simulink library "tqd"  (R2021b)
settings: Solver=VariableStepAuto  StartTime=0.0  StopTime=10.0  RelTol=1e-3
undefined symbols (not defined in the file): ATQD_AfterTqMinGain_X_Deg, ATQD_APSCreepBaseTqD_X_kph, ATQD_APSCreepBaseTqD_Y_Deg, ATQD_APSCreepBaseTqR_X_kph, ATQD_APSCreepBaseTqR_Y_Deg, ATQD_APSCreepIterm_X_kph, ATQD_APSCreepIterm_Y_kph, ATQD_APSCreepPterm_X_kph, ATQD_APSCreepPterm_Y_kph, ATQD_APSDecReq_X_kph, ATQD_APSDecReq_Y_mps2, ATQD_APSDecReqCMD_X_kph, ATQD_APSDecReqTs_X_pct, ATQD_APSDecTimeGain_X_Deg, ATQD_APSDecTimeGain_Y_s, ATQD_APSReqLowSpd_X_Deg, ATQD_AutoHoldReleaseBPS_X_Deg, ATQD_AWDLoadTrqnsGain_X_kg, ATQD_AWDLoadTrqnsGain_Y_pct, ATQD_BOSEnBPSPosn_X_kph, ATQD_BOSMap_X_rpm, ATQD_BOSMap_Y_pct, ATQD_CreepBaseTqD_X_kph, ATQD_CreepBaseTqD_Y_Deg, ATQD_CreepBaseTqR_X_kph, ATQD_CreepBaseTqR_Y_Deg, ATQD_CreepBPSDisPosn_X_Deg, ATQD_CreepBPSDisPosnR_X_Deg, ATQD_CreepBPSEnPosn_X_Deg, ATQD_CreepBPSEnPosnR_X_Deg, ATQD_CreepDeltaTq_X_kph, ATQD_CreepIterm_X_kph, ATQD_CreepIterm_Y_kph, ATQD_CreepItermMaxLimit_X_pct, ATQD_CreepPreloadTime_X_kph, ATQD_CreepPreloadTq_X_kph, ATQD_CreepPreloadTq_Y_s, ATQD_CreepProtTq_X_Deg, ATQD_CreepPterm_X_kph, ATQD_CreepPterm_Y_kph, ATQD_CreepRrTqSpRat_X_rpm, ATQD_CreepRrTqSpRat_Y_Nm, ATQD_CreepTargetSpdD_X_pct, ATQD_CreepTargetSpdR_X_pct, ATQD_ECOTqMapD_X_rpm, ATQD_ECOTqMapD_Y_pct, ATQD_EMTqMapD_X_rpm, ATQD_EMTqMapD_Y_pct, ATQD_EOPDTqMapDCon_X_rpm, ATQD_EOPDTqMapDCon_Y_Deg, ATQD_EscapeModePedTq_X_pct, ATQD_EscapeModePedTq_Y_rpm, ATQD_EscapeModePedTqFr_X_pct, ATQD_EscapeModePedTqFr_Y_rpm, ATQD_EstInitVehWeight_X_c, ATQD_FAfterTqCMDGain_X_rpm, ATQD_FAfterTqCMDGain_Y_pct, ATQD_FrLossMAPLowV_X_rpm, ATQD_FrLossMAPLowV_Y_Nm, ATQD_FrMotActReduce_X_rpm ... (+772)
libraries: simulink x211, hcu_lib x179, tqr x3
(part 6 of 28)

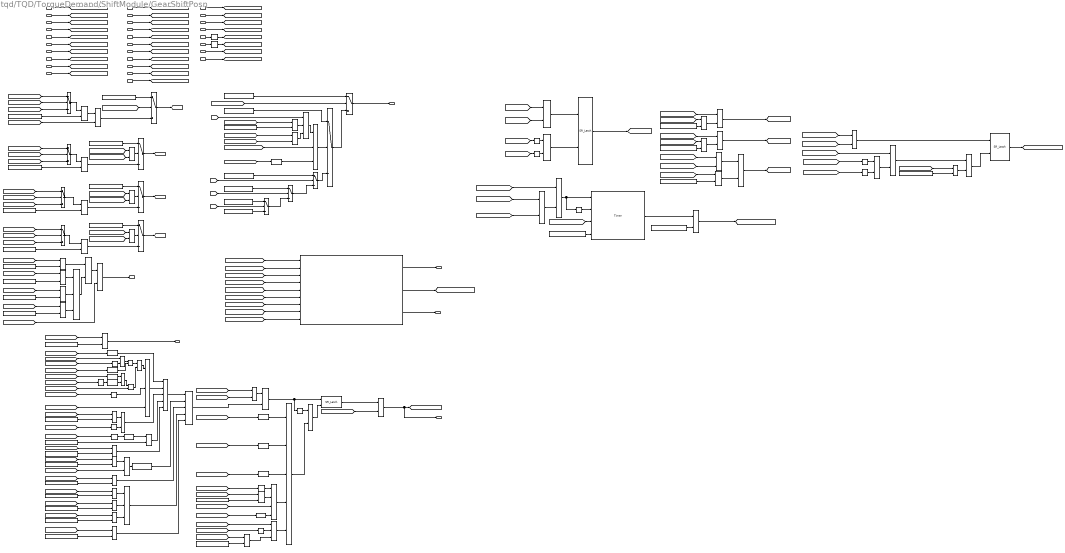
== system tqd/TQD/TorqueDemand/ShiftModule/GearShiftPosn ==
  note: Failsafe for Shifter PButton fail
  VTQD_ShifterHandleCmd_enum : Inport
  VPMM_PowerSta_enum : Inport  Port=2
  VINP_DrDoorSW_flg : Inport  Port=3
  VVMC_APSShiftPosnReq_enum : Inport  Port=4
  VVMC_APSActive_flg : Inport  Port=5
  VINP_DriverSeatBeltCmd_flg : Inport  Port=6
  VINP_SeatSW_flg : Inport  Port=7
  VTQD_EPBCarWashMode_flg : Inport  Port=8
  VTQD_VehActSpd_kph : Inport  Port=9
  VINP_ChrgPlugSta_enum : Inport  Port=10
  VTQD_GearActualPosn_enum : Inport  Port=11
  VTQD_AfterAvailableTqDemFr_Nm : Inport  Port=12
  VTQD_AfterAvailableTqDemRr_Nm : Inport  Port=13
  VTQR_NoABSFEDUWhlTqReq_Nm : Inport  Port=14
  VTQR_NoABSREDUWhlTqReq_Nm : Inport  Port=15
  task_time_s : Inport  Port=16
  VINP_DOASta_flg : Inport  Port=17
  VTQD_IVIPwrLock_flg : Inport  Port=18
  VTQD_BrkSwSta_flg : Inport  Port=19
  VTQD_OPDHoldAllowPark_flg : Inport  Port=20
  VINP_CAASSta_enum : Inport  Port=21
  VDDM_VCURAPSErrLv2_flg : Inport  Port=22
  VDDM_VCURAPSErrLv3_flg : Inport  Port=23
  VINP_APSStaSystem_enum : Inport  Port=24
  VDDM_Shifter1Err_flg : Inport  Port=25
  SWC_RegenUp : Inport  Port=26
  SWC_RegenDown : Inport  Port=27
  VDDM_ShifterSigErrCFS_flg : Inport  Port=28
  VTQD_ShifterFailsta_enum : Inport  Port=29
  AND{,1,6..9} (6 alike) : Logic  AllPortsSameDT=off  OutDataTypeStr=boolean
  AND2 : Logic  Inputs=4  AllPortsSameDT=off  OutDataTypeStr=boolean
  AND3 : Logic  Operator=OR  AllPortsSameDT=off  OutDataTypeStr=boolean
  AND4 : Logic  Inputs=3  AllPortsSameDT=off  OutDataTypeStr=boolean
  AND5 : Logic  Inputs=5  AllPortsSameDT=off  OutDataTypeStr=boolean
  Constant : Constant  Value=ENUM_GEARSHIFTCMD_R
  Constant1 : Constant  Value=ENUM_POWERSTA_READY
  Constant10 : Constant  Value=KTQD_OPDHoldAllowGearPSW_flg
  Constant11 : Constant  Value=ENUM_CAASSTA_SHIFTGEARTOP
  Constant12 : Constant  Value=ENUM_SHIFTCOMMAND_D
  Constant13 : Constant  Value=ENUM_SHIFTCOMMAND_N
  Constant14 : Constant  Value=ENUM_PWRSTASW_READY
  Constant15 : Constant  Value=ENUM_SHIFTCOMMAND_P
  Constant16 : Constant  Value=ENUM_CHRGPLUGSTA_NONE
  Constant17 : Constant  Value=ENUM_POWERSTA_STANDBY
  Constant18 : Constant  Value=ENUM_POWERSTA_ON
  Constant19 : Constant  Value=ENUM_POWERSTA_READY
  Constant2 : Constant  Value=ENUM_GEARSHIFTCMD_N
  Constant20 : Constant  Value=ENUM_APSSYSTEMSTA_REMOTEACTIVE
  Constant21 : Constant  Value=ENUM_APSSYSTEMSTA_REMOTEACTIVE
  Constant22 : Constant  Value=ENUM_CHRGPLUGSTA_NONE
  Constant23 : Constant  Value=ENUM_PWRSTASW_STANDBY
  Constant24 : Constant  Value=ENUM_PWRSTASW_ON
  Constant25 : Constant  Value=ENUM_PWRSTASW_READY
  Constant26 : Constant  Value=KTQD_ForcePLimitSpd_kph
  Constant27 : Constant  Value=KTQD_ShifterFail2P_s
  Constant28 : Constant  Value=KTQD_ShifterFail2P_s
  Constant29 : Constant  Value=KTQD_ForcePLimitSpd_kph
  Constant3 : Constant  Value=ENUM_GEARSHIFTCMD_P
  Constant30 : Constant  Value=ENUM_SHIFTERERRSTA_PBUTTONFAILURE
  Constant31 : Constant  Value=ENUM_SHIFTERERRSTA_HALLFAILURE
  Constant{5,32..34} (4 alike) : Constant  Value=FALSE
  Constant35 : Constant  Value=ENUM_SHIFTERERRSTA_SHIFTERFAILURE
  Constant36 : Constant  Value=ENUM_SHIFTCOMMAND_R
  Constant4 : Constant  Value=ENUM_GEARSHIFTCMD_D
  Constant6 : Constant  Value=ENUM_GEARSHIFTCMD_NONE
  Constant7 : Constant  Value=ENUM_GEARSHIFTCMD_P
  Constant8 : Constant  Value=ENUM_SHIFTCOMMAND_P
  Constant9 : Constant  Value=KTQD_DriveProtVehSpdGain_kph
  Delay{,1..3} (4 alike) : Delay  DelayLength=1
  Detect Change : simulink/Logic and Bit Operations/Detect Change  vinit=0  OutDataTypeStr=boolean
  Detect Change1 : simulink/Logic and Bit Operations/Detect Change  vinit=0  OutDataTypeStr=boolean
  Detect Decrease1 : simulink/Logic and Bit Operations/Detect Decrease  vinit=0.0  OutDataTypeStr=boolean
  Detect Increase{,1..6} (7 alike) : simulink/Logic and Bit Operations/Detect Increase  vinit=0.0  OutDataTypeStr=boolean
  Drive Protection : Subsystem
  Equal{,1..7,9..10,12..13,15..16,18..20} (17 alike) : RelationalOperator  Operator===  OutDataTypeStr=boolean  RndMeth=Simplest
  Equal11 : RelationalOperator  Operator=~=  OutDataTypeStr=boolean  RndMeth=Simplest
  Equal14 : RelationalOperator  Operator=~=  OutDataTypeStr=boolean  RndMeth=Simplest
  Equal8 : RelationalOperator  Operator=<=  OutDataTypeStr=boolean  RndMeth=Simplest
  Latch : hcu_lib/Basic_Blocks/Latch
  Logical Operator{,1,7,10..12,14,20,23} (9 alike) : Logic  AllPortsSameDT=off  OutDataTypeStr=boolean
      Logical Operator20 settings: AttributesFormatString=%<Operator>
  Logical Operator{8..9,13,16..19,24} (8 alike) : Logic  Operator=OR  AllPortsSameDT=off  OutDataTypeStr=boolean
      Logical Operator24 settings: AttributesFormatString=%<Operator>
  Logical Operator{4,15,21..22} (4 alike) : Logic  Operator=NOT  AllPortsSameDT=off  OutDataTypeStr=boolean
  Logical Operator2 : Logic  Inputs=3  AllPortsSameDT=off  OutDataTypeStr=boolean
  Logical Operator3 : Logic  Operator=OR  Inputs=3  AllPortsSameDT=off  OutDataTypeStr=boolean
  Logical Operator6 : Logic  Inputs=3  AllPortsSameDT=off  OutDataTypeStr=boolean
  NOT{,2..7} (7 alike) : Logic  Operator=NOT  AllPortsSameDT=off  OutDataTypeStr=boolean
  OR : Logic  Operator=OR  Inputs=3  AllPortsSameDT=off  OutDataTypeStr=boolean
  OR1 : Logic  Operator=OR  Inputs=5  AllPortsSameDT=off  OutDataTypeStr=boolean
  OR{2..6,9..10} (7 alike) : Logic  Operator=OR  AllPortsSameDT=off  OutDataTypeStr=boolean
  OR7 : Logic  Operator=OR  Inputs=5  AllPortsSameDT=off  OutDataTypeStr=boolean
  OR8 : Logic  Operator=OR  Inputs=3  AllPortsSameDT=off  OutDataTypeStr=boolean
  Relational Operator1 : RelationalOperator  Operator===  OutDataTypeStr=boolean  RndMeth=Simplest
  Relational Operator2 : RelationalOperator  Operator=<=  OutDataTypeStr=boolean  RndMeth=Simplest
  Relational Operator3 : RelationalOperator  OutDataTypeStr=boolean  RndMeth=Simplest
  Relational Operator4 : RelationalOperator  Operator=<=  OutDataTypeStr=boolean  RndMeth=Simplest
  Relational Operator5 : RelationalOperator  Operator=~=  OutDataTypeStr=boolean  RndMeth=Simplest
  SR_Latch : hcu_lib/Basic_Blocks/SR_Latch
  SR_Latch1 : hcu_lib/Basic_Blocks/SR_Latch
  SR_Latch3 : hcu_lib/Basic_Blocks/SR_Latch
  Switch{,1..4,7} (6 alike) : Switch  Criteria=u2 ~= 0
      Switch1 settings: AttributesFormatString=%<Criteria>
      Switch2 settings: AttributesFormatString=%<Criteria>
      Switch3 settings: AttributesFormatString=%<Criteria>
      Switch4 settings: AttributesFormatString=%<Criteria>
  Switch{5..6,8,10..13} (7 alike) : Switch  Criteria=u2 > Threshold
  Timer : hcu_lib/Basic_Blocks/Timer
  VTQD_GearShiftCMD_enum : Outport
  VTQD_PwrStaAllowPN_flg : Outport  Port=2
  VTQD_PwrStaAllowDR_flg : Outport  Port=3
  VTQD_DriveProtRemove_flg : Outport  Port=4
  VTQD_DriveProtEn_flg : Outport  Port=5
  VTQD_ForceP_flg : Outport  Port=6
  wires:
  Switch2/1 -> Switch4/3
  Constant2/1 -> Switch4/1
  Switch1/1 -> Switch2/3
  [P] -> Switch2/2
  Constant3/1 -> Switch2/1
  Switch3/1 -> Switch1/3
  Constant/1 -> Switch3/1
  Constant4/1 -> Switch1/1
  [R] -> Switch3/2
  [D] -> Switch1/2
  VTQD_ShifterHandleCmd_enum/1 -> [VTQD_ShifterHandleCmd_enum]
  Constant19/1 -> Equal6/2
  [VPMM_PowerSta_enum] -> Equal6/1
  [VPMM_PowerSta_enum] -> Equal5/1
  [VPMM_PowerSta_enum] -> Equal4/1
  Constant17/1 -> Equal4/2
  Constant18/1 -> Equal5/2
  VPMM_PowerSta_enum/1 -> [VPMM_PowerSta_enum]
  Equal5/1 -> OR/2
  Equal4/1 -> OR/1
  Equal6/1 -> OR/3
  [VPMM_PowerSta_enum] -> Equal7/1
  Constant1/1 -> Equal7/2
  Equal7/1 -> VTQD_PwrStaAllowDR_flg/1  "VTQD_PwrStaAllowDR_flg"
  Constant6/1 -> Switch3/3
  Switch/1 -> VTQD_GearShiftCMD_enum/1  "VTQD_GearShiftCMD_enum"
  Switch4/1 -> Switch/3
  VINP_DrDoorSW_flg/1 -> [VINP_DrDoorSW_flg]
  [VTQD_ForceP_flg] -> Switch/2
  Constant7/1 -> Switch/1
  VVMC_APSShiftPosnReq_enum/1 -> [VVMC_APSShiftPosnReq_enum]
  VVMC_APSActive_flg/1 -> [VVMC_APSActive_flg]
  VINP_SeatSW_flg/1 -> [VINP_SeatSW_flg]
  VINP_DriverSeatBeltCmd_flg/1 -> [VINP_DriverSeatBeltCmd_flg]
  VTQD_EPBCarWashMode_flg/1 -> [VTQD_EPBCarWashMode_flg]
  VTQD_VehActSpd_kph/1 -> [VTQD_VehActSpd_kph]
  VINP_ChrgPlugSta_enum/1 -> [VINP_ChrgPlugSta_enum]
  VTQR_NoABSREDUWhlTqReq_Nm/1 -> [VTQR_NoABSREDUWhlTqReq_Nm]
  VTQD_AfterAvailableTqDemFr_Nm/1 -> [VTQD_AfterAvailableTqDemFr_Nm]
  VTQD_GearActualPosn_enum/1 -> [VTQD_GearActualPosn_enum]
  VTQR_NoABSFEDUWhlTqReq_Nm/1 -> [VTQR_NoABSFEDUWhlTqReq_Nm]
  VTQD_AfterAvailableTqDemRr_Nm/1 -> [VTQD_AfterAvailableTqDemRr_Nm]
  task_time_s/1 -> [task_time_s]
  OR6/1 -> Logical Operator/1
  Logical Operator1/1 -> OR10/2
  [VTQD_EPBCarWashMode_flg] -> NOT4/1
  [VPMM_PowerSta_enum] -> Equal15/1
  [VTQD_VehActSpd_kph] -> Relational Operator2/1
  Logical Operator/1 -> OR10/1
  Detect Increase3/1 -> OR9/2
  [VINP_DrDoorSW_flg] -> Logical Operator1/2
  [VINP_SeatSW_flg] -> NOT5/1
  [VINP_DrDoorSW_flg] -> Detect Increase1/1
  OR9/1 -> Logical Operator1/1
  Detect Increase2/1 -> OR9/1
  Constant16/1 -> Equal14/2
  NOT5/1 -> Detect Increase3/1
  [VINP_DriverSeatBeltCmd_flg] -> Detect Increase2/1
  Equal12/1 -> OR8/2
  OR10/1 -> AND4/1
  AND4/1 -> OR7/2
  Equal15/1 -> OR8/1
  Constant23/1 -> Equal15/2
  Constant25/1 -> Equal13/2
  Detect Increase1/1 -> Logical Operator/2
  [VTQD_EPBCarWashMode_flg] -> Detect Decrease1/1
  Constant26/1 -> Relational Operator2/2
  [VPMM_PowerSta_enum] -> Equal13/1
  NOT4/1 -> AND4/2
  Constant24/1 -> Equal12/2
  Equal13/1 -> OR8/3
  [VINP_ChrgPlugSta_enum] -> Equal14/1
  OR7/1 -> AND5/1
  NOT3/1 -> OR6/2
  Detect Decrease1/1 -> OR7/1
  [VINP_DriverSeatBeltCmd_flg] -> OR6/1
  [VINP_SeatSW_flg] -> NOT3/1
  [VPMM_PowerSta_enum] -> Equal12/1
  VINP_DOASta_flg/1 -> [VINP_DOASta_flg]
  [VINP_DOASta_flg] -> AND4/3
  Constant9/1 -> Equal8/2
  [VTQD_VehActSpd_kph] -> Equal8/1
  [VTQD_EPBCarWashMode_flg] -> Detect Increase/1
  Detect Increase/1 -> Logical Operator3/3
  [N] -> Logical Operator2/1
  Logical Operator2/1 -> Logical Operator3/1
  Logical Operator3/1 -> Switch4/2
  [task_time_s] -> Drive Protection/8(task_time_s)  "task_time_s"
  [VTQD_VehActSpd_kph] -> Drive Protection/3(VTQD_VehActSpd_kph)
  [VTQD_AfterAvailableTqDemRr_Nm] -> Drive Protection/7(VTQD_AfterAvailableTqDemRr_Nm)
  Drive Protection/1(VTQD_DriveProtRemove_flg) -> VTQD_DriveProtRemove_flg/1
  [VTQD_AfterAvailableTqDemFr_Nm] -> Drive Protection/4(VTQD_AfterAvailableTqDemFr_Nm)
  [VTQR_NoABSREDUWhlTqReq_Nm] -> Drive Protection/5(VTQR_NoABSREDUWhlTqReq_Nm)
  [VTQR_NoABSFEDUWhlTqReq_Nm] -> Drive Protection/6(VTQR_NoABSFEDUWhlTqReq_Nm)
  [VTQD_ShifterHandleCmd_enum] -> Drive Protection/1(VTQD_ShifterHandleCmd_enum)
  Drive Protection/2(VTQD_DriveProtToPsnN_flg) -> [VTQD_DriveProtToPsnN_flg]
  [VTQD_GearActualPosn_enum] -> Drive Protection/2(VTQD_GearActualPosn_enum)
  VTQD_IVIPwrLock_flg/1 -> [VTQD_IVIPwrLock_flg]
  [VTQD_DriveProtToPsnN_flg] -> Logical Operator3/2
  Drive Protection/3(VTQD_DriveProtEn_flg) -> VTQD_DriveProtEn_flg/1
  [VTQD_IVIPwrLock_flg] -> OR2/2
  SR_Latch1/1 -> OR2/1
  OR2/1 -> VTQD_ForceP_flg/1, [VTQD_ForceP_flg]  "VTQD_ForceP_flg"
  [VPMM_PowerSta_enum] -> Equal3/1
  Latch/1 -> AND5/2
  Constant14/1 -> Equal3/2
  Relational Operator2/1 -> AND5/3
  OR8/1 -> AND5/4
  Equal8/1 -> Logical Operator2/2
  VTQD_BrkSwSta_flg/1 -> [VTQD_BrkSwSta_flg]
  [VTQD_BrkSwSta_flg] -> Drive Protection/9(VTQD_BrkSwSta_flg)
  OR3/1 -> Logical Operator2/3
  [VTQD_BrkSwSta_flg] -> OR3/1
  [VVMC_APSActive_flg] -> OR3/2
  VTQD_OPDHoldAllowPark_flg/1 -> [VTQD_OPDHoldAllowPark_flg]
  AND/1 -> OR7/4
  Detect Increase6/1 -> AND/1
  Constant10/1 -> AND/2
  [VTQD_OPDHoldAllowPark_flg] -> Delay/1
  Delay/1 -> Detect Increase6/1
  VINP_CAASSta_enum/1 -> [VINP_CAASSta_enum]
  [VINP_CAASSta_enum] -> Equal10/1
  Equal10/1 -> OR7/5
  Constant11/1 -> Equal10/2
  VDDM_VCURAPSErrLv3_flg/1 -> [VDDM_VCURAPSErrLv3_flg]
  VINP_APSStaSystem_enum/1 -> [VINP_APSStaSystem_enum]
  VDDM_VCURAPSErrLv2_flg/1 -> [VDDM_VCURAPSErrLv2_flg]
  [VVMC_APSActive_flg] -> Logical Operator7/1
  [VDDM_VCURAPSErrLv3_flg] -> Logical Operator7/2
  Logical Operator7/1 -> AND3/1
  AND5/1 -> AND3/2
  [VDDM_VCURAPSErrLv3_flg] -> Logical Operator4/1
  [VVMC_APSActive_flg] -> Detect Increase5/1
  [VINP_APSStaSystem_enum] -> Relational Operator1/1
  Logical Operator6/1 -> OR1/5
  Delay1/1 -> AND2/1
  Constant21/1 -> Relational Operator1/2
  [VTQD_ShifterHandleCmd_enum] -> Detect Change/1
  AND2/1 -> OR1/4
  Detect Increase5/1 -> OR1/3
  Equal11/1 -> AND2/2
  Detect Change1/1 -> AND2/4
  Relational Operator1/1 -> Logical Operator6/3
  [VVMC_APSShiftPosnReq_enum] -> Equal11/1
  [VTQD_EPBCarWashMode_flg] -> Detect Increase4/1
  [VDDM_VCURAPSErrLv2_flg] -> Logical Operator6/1
  OR1/1 -> AND1/2
  [VTQD_ForceP_flg] -> Delay1/1
  AND1/1 -> SR_Latch1/2
  Detect Increase4/1 -> OR1/2
  Detect Change/1 -> OR1/1
  [VVMC_APSShiftPosnReq_enum] -> Detect Change1/1
  Constant15/1 -> Equal11/2
  Logical Operator4/1 -> Logical Operator6/2
  [VVMC_APSActive_flg] -> AND2/3
  AND3/1 -> SR_Latch1/1, NOT/1
  NOT/1 -> AND1/1
  OR/1 -> AND6/2
  [VINP_ChrgPlugSta_enum] -> Equal16/1
  Constant22/1 -> Equal16/2
  Equal16/1 -> AND6/1
  AND6/1 -> OR4/1
  [VTQD_EPBCarWashMode_flg] -> OR4/2
  OR4/1 -> VTQD_PwrStaAllowPN_flg/1  "VTQD_PwrStaAllowPN_flg"
  Equal14/1 -> AND7/1
  [VTQD_EPBCarWashMode_flg] -> NOT2/1
  NOT2/1 -> AND7/2
  AND7/1 -> OR7/3
  Constant8/1 -> Equal/2
  Equal1/1 -> Switch11/3
  Switch8/1 -> Equal2/1
  Switch10/1 -> [P]
  [ShifterHall_Fail] -> Logical Operator17/1
  Constant33/1 -> Switch12/1
  [VVMC_APSShiftPosnReq_enum] -> Switch6/1
  [VVMC_APSActive_flg] -> Switch7/2
  [Shifter_Fail] -> Logical Operator18/2
  Switch13/1 -> [N]
  Constant13/1 -> Equal9/2
  [VVMC_APSActive_flg] -> Switch8/2
  [VVMC_APSShiftPosnReq_enum] -> Switch8/1
  [VVMC_APSActive_flg] -> Switch6/2
  Equal9/1 -> Switch13/3
  Logical Operator8/1 -> Switch11/2
  [Shifter_Fail] -> Logical Operator17/2
  Switch7/1 -> Equal9/1
  [VTQD_ShifterHandleCmd_enum] -> Switch5/3
  Constant5/1 -> Switch10/1
  Switch12/1 -> [D]
  [VVMC_APSShiftPosnReq_enum] -> Switch5/1
  Equal2/1 -> Switch12/3
  [VTQD_ShifterHandleCmd_enum] -> Switch6/3
  [VVMC_APSShiftPosnReq_enum] -> Switch7/1
  Constant12/1 -> Equal2/2
  Switch5/1 -> Equal/1
  Constant32/1 -> Switch11/1
  [ShifterHall_Fail] -> Logical Operator8/1
  Switch11/1 -> [R]
  Constant36/1 -> Equal1/2
  [VTQD_ShifterFail2P_flg] -> Logical Operator19/2
  [VTQD_ShifterHandleCmd_enum] -> Switch8/3
  [ShifterHall_Fail] -> Logical Operator18/1
  [VTQD_ShifterHandleCmd_enum] -> Switch7/3
  Equal/1 -> Logical Operator19/1
  Logical Operator19/1 -> Switch10/3
  Constant34/1 -> Switch13/1
  Logical Operator18/1 -> Switch13/2
  [VTQD_ShifterPBackUpCmd_flg] -> Switch10/2
  Switch6/1 -> Equal1/1
  [Shifter_Fail] -> Logical Operator8/2
  Logical Operator17/1 -> Switch12/2
  [VVMC_APSActive_flg] -> Switch5/2
  Logical Operator15/1 -> Timer/2
  [Shifter_Fail] -> Logical Operator16/2
  SR_Latch/1 -> [PRESS_BOTH]
  Constant29/1 -> Relational Operator4/2
  Logical Operator22/1 -> Logical Operator20/2
  AND9/1 -> SR_Latch/2
  Logical Operator13/1 -> Logical Operator14/1
  [VDDM_ShifterSigErrCFS_flg] -> Logical Operator12/1
  [VDDM_Shifter1Err_flg] -> Logical Operator13/2
  [SWC_RegenDown] -> NOT7/1
  Logical Operator21/1 -> Logical Operator20/1
  Logical Operator14/1 -> [Shifter_Fail]
  NOT7/1 -> AND9/2
  [task_time_s] -> Timer/3
  Relational Operator3/1 -> [VTQD_ShifterFail2P_flg]  "VTQD_ShifterFail2P_flg"
  [PRESS_BOTH] -> Logical Operator10/1
  Constant31/1 -> Equal19/2
  Logical Operator20/1 -> Logical Operator24/2
  [PRESS_BOTH] -> Logical Operator24/1
  Logical Operator12/1 -> [ShifterHall_Fail]
  [SWC_RegenUp] -> NOT6/1
  [Shifter_Fail] -> Logical Operator9/1
  [VTQD_ShifterFailsta_enum] -> Equal18/1
  Logical Operator16/1 -> SR_Latch3/1
  Logical Operator23/1 -> SR_Latch3/2
  Logical Operator24/1 -> Logical Operator23/1
  Relational Operator4/1 -> Logical Operator23/2
  [SWC_RegenDown] -> AND8/2
  [ShifterPButton_Fail] -> Logical Operator9/2
  Constant27/1 -> Timer/4
  Equal18/1 -> Logical Operator11/2
  Equal19/1 -> Logical Operator12/2
  [VDDM_ShifterSigErrCFS_flg] -> Logical Operator13/1
  [VDDM_ShifterSigErrCFS_flg] -> Logical Operator11/1
  AND8/1 -> SR_Latch/1
  Constant28/1 -> Relational Operator3/2
  Constant30/1 -> Equal18/2
  Timer/1 -> Relational Operator3/1
  Equal20/1 -> Logical Operator14/2
  Logical Operator9/1 -> Logical Operator10/2
  SR_Latch3/1 -> [VTQD_ShifterPBackUpCmd_flg]
  [ShifterPButton_Fail] -> Logical Operator16/1
  Logical Operator11/1 -> [ShifterPButton_Fail]
  [SWC_RegenUp] -> AND8/1
  [VTQD_ShifterFailsta_enum] -> Equal19/1
  Constant35/1 -> Equal20/2
  [VTQD_VehActSpd_kph] -> Relational Operator4/1
  NOT6/1 -> AND9/1
  [VTQD_ShifterFailsta_enum] -> Equal20/1
  Logical Operator10/1 -> Logical Operator15/1, Timer/1
  [VDDM_Shifter1Err_flg] -> Logical Operator22/1
  [VDDM_ShifterSigErrCFS_flg] -> Logical Operator21/1
  Constant20/1 -> Relational Operator5/2
  [VINP_APSStaSystem_enum] -> Relational Operator5/1
  Relational Operator5/1 -> AND5/5
  VDDM_ShifterSigErrCFS_flg/1 -> [VDDM_ShifterSigErrCFS_flg]
  Delay2/1 -> [SWC_RegenUp]
  SWC_RegenUp/1 -> Delay2/1
  Delay3/1 -> [SWC_RegenDown]
  SWC_RegenDown/1 -> Delay3/1
  VDDM_Shifter1Err_flg/1 -> [VDDM_Shifter1Err_flg]
  VTQD_ShifterFailsta_enum/1 -> [VTQD_ShifterFailsta_enum]
  [VINP_DOASta_flg] -> OR5/2
  Equal3/1 -> OR5/1
  OR5/1 -> Latch/1

== system tqd/TQD/TorqueDemand/ShiftModule/P_Button_State_Judge ==
  VTQD_ShifterHandleCmd_enum : Inport
  VVMC_APSActive_flg : Inport  Port=2
  VVMC_APSShiftPosnReq_enum : Inport  Port=3
  VTQD_ParkRequest_flg : Inport  Port=4
  VINP_EPBSta_enum : Inport  Port=5
  AND : Logic  AllPortsSameDT=off  OutDataTypeStr=boolean
  AND1 : Logic  Operator=OR  AllPortsSameDT=off  OutDataTypeStr=boolean
  Constant1 : Constant  Value=ENUM_PBUTTON_RELEASED
  Constant10 : Constant  Value=ENUM_EPBSTA_APPLIED
  Constant12 : Constant  Value=ENUM_SHIFTCOMMAND_D
  Constant15 : Constant  Value=ENUM_SHIFTCOMMAND_N
  Constant2 : Constant  Value=ENUM_PBUTTON_PRESSED
  Constant3 : Constant  Value=ENUM_PBUTTON_INVALID
  Constant4 : Constant  Value=ENUM_SHIFTCOMMAND_NONE
  Constant5 : Constant  Value=ENUM_SHIFTCOMMAND_P
  Constant6 : Constant  Value=ENUM_SHIFTCOMMAND_P
  Constant7 : Constant  Value=ENUM_PBUTTON_PRESSED
  Constant8 : Constant  Value=ENUM_SHIFTCOMMAND_R
  Constant9 : Constant  Value=ENUM_EPBSTA_APPLIED
  Detect Decrease : simulink/Logic and Bit Operations/Detect Decrease  vinit=boolean(0)  OutDataTypeStr=boolean
  Detect Decrease1 : simulink/Logic and Bit Operations/Detect Decrease  vinit=boolean(0)  OutDataTypeStr=boolean
  Detect Increase : simulink/Logic and Bit Operations/Detect Increase  vinit=boolean(0)  OutDataTypeStr=boolean
  Detect Increase1 : simulink/Logic and Bit Operations/Detect Increase  vinit=boolean(0)  OutDataTypeStr=boolean
  Equal{,1..7} (8 alike) : RelationalOperator  Operator===  OutDataTypeStr=boolean  RndMeth=Simplest
  Logical Operator : Logic  Operator=OR  Inputs=4  AllPortsSameDT=off  OutDataTypeStr=boolean
  NOT : Logic  Operator=NOT  AllPortsSameDT=off  OutDataTypeStr=boolean
  OR : Logic  Operator=OR  AllPortsSameDT=off  OutDataTypeStr=boolean
  OR1 : Logic  Operator=OR  Inputs=3  AllPortsSameDT=off  OutDataTypeStr=boolean
  SR_Latch : hcu_lib/Basic_Blocks/SR_Latch
  SR_Latch1 : hcu_lib/Basic_Blocks/SR_Latch
  Switch1 : Switch  Criteria=u2 ~= 0
      settings: AttributesFormatString=%<Criteria>
  Switch2 : Switch  Criteria=u2 ~= 0
      settings: AttributesFormatString=%<Criteria>
  Switch4 : Switch  Criteria=u2 ~= 0
      settings: AttributesFormatString=%<Criteria>
  VTQD_PButtonSta_enum : Outport
  wires:
  VTQD_ShifterHandleCmd_enum/1 -> [VTQD_ShifterHandleCmd_enum]
  Equal/1 -> [P]
  Constant12/1 -> Equal2/2
  [VTQD_ShifterHandleCmd_enum] -> Equal1/1
  Constant8/1 -> Equal1/2
  [VTQD_ShifterHandleCmd_enum] -> Equal/1
  Equal2/1 -> Logical Operator/3
  Constant15/1 -> Equal3/2
  Equal3/1 -> Logical Operator/2
  Equal1/1 -> Logical Operator/1
  Constant5/1 -> Equal/2
  [VTQD_ShifterHandleCmd_enum] -> Equal3/1
  [VTQD_ShifterHandleCmd_enum] -> Equal2/1
  Logical Operator/1 -> [RND]
  [RND] -> Switch4/2
  [P] -> Switch1/2
  Constant1/1 -> Switch4/1
  Switch1/1 -> Switch4/3
  Constant2/1 -> Switch1/1
  Constant3/1 -> Switch1/3
  [VTQD_ShifterHandleCmd_enum] -> Equal4/1
  Constant4/1 -> Equal4/2
  Equal4/1 -> Logical Operator/4
  Switch4/1 -> Switch2/3
  VVMC_APSActive_flg/1 -> [VVMC_APSActive_flg]
  VVMC_APSShiftPosnReq_enum/1 -> [VVMC_APSShiftPosnReq_enum]
  Switch2/1 -> VTQD_PButtonSta_enum/1  "VTQD_PButtonSta_enum"
  [VVMC_APSShiftPosnReq_enum] -> Equal5/1
  Constant6/1 -> Equal5/2
  [VVMC_APSActive_flg] -> AND/1
  Equal5/1 -> AND/2
  Constant7/1 -> Switch2/1
  VTQD_ParkRequest_flg/1 -> [VTQD_ParkRequest_flg]
  AND1/1 -> Switch2/2
  SR_Latch/1 -> AND1/1
  [VTQD_ParkRequest_flg] -> Detect Decrease/1, Detect Increase/1
  [VINP_EPBSta_enum] -> Equal6/1
  Detect Increase/1 -> SR_Latch/1
  Constant9/1 -> Equal6/2
  VINP_EPBSta_enum/1 -> [VINP_EPBSta_enum]
  OR/1 -> SR_Latch/2
  Equal6/1 -> OR/2
  Detect Decrease/1 -> OR/1
  AND/1 -> Detect Decrease1/1, Detect Increase1/1
  Detect Increase1/1 -> SR_Latch1/1
  [VINP_EPBSta_enum] -> Equal7/1
  Constant10/1 -> Equal7/2
  OR1/1 -> SR_Latch1/2
  SR_Latch1/1 -> AND1/2
  Equal7/1 -> OR1/3
  Detect Decrease1/1 -> OR1/1
  NOT/1 -> OR1/2
  [VVMC_APSActive_flg] -> NOT/1

== system tqd/TQD/TorqueDemand/ShiftModule/SR_Latch1 ==
  set : Inport
  reset : Inport  Port=2
  Logical Operator : Logic  AllPortsSameDT=off  OutDataTypeStr=boolean
  Logical Operator1 : Logic  Operator=NOT  AllPortsSameDT=off  OutDataTypeStr=boolean
  Switch1 : Switch  Criteria=u2 ~= 0  Threshold=0.5
      settings: AttributesFormatString=<Criteria=%<Criteria>>
  Switch2 : Switch  Criteria=u2 ~= 0  Threshold=0.5
      settings: AttributesFormatString=<Criteria=%<Criteria>>
  Unit Delay : UnitDelay  SampleTime=-1  HasFrameUpgradeWarning=on
  latched : Outport
  wires:
  Switch1/1 -> Unit Delay/1, latched/1
  set/1 -> Switch1/1, Logical Operator/1
  reset/1 -> Switch2/2, Logical Operator1/1
  Unit Delay/1 -> Switch2/3
  Switch2/1 -> Switch1/3
  Logical Operator/1 -> Switch1/2
  Logical Operator1/1 -> Logical Operator/2, Switch2/1

== system tqd/TQD/TorqueDemand/Signal_convert/AWDMCUReadyExt_flg ==
  VINP_FrMCUErr_enum : Inport
  VINP_RrMCUErr_enum : Inport  Port=2
  Action Port : ActionPort
  Constant : Constant  Value=ENUM_MCUWARN_LV0
  Constant1 : Constant  Value=ENUM_MCUWARN_NOERROR
  Constant2 : Constant  Value=ENUM_MCUWARN_LV0
  Constant3 : Constant  Value=ENUM_MCUWARN_NOERROR
  Equal{,1..3} (4 alike) : RelationalOperator  Operator===  OutDataTypeStr=boolean  RndMeth=Simplest
  Logical Operator : Logic  Operator=OR  AllPortsSameDT=off  OutDataTypeStr=boolean
  Logical Operator1 : Logic  Operator=OR  AllPortsSameDT=off  OutDataTypeStr=boolean
  Logical Operator2 : Logic  AllPortsSameDT=off  OutDataTypeStr=boolean
  VTQD_AWDMCUReadyExt_flg : Outport
  wires:
  Logical Operator2/1 -> VTQD_AWDMCUReadyExt_flg/1
  Equal1/1 -> Logical Operator/2
  Equal/1 -> Logical Operator/1
  Constant1/1 -> Equal1/2
  VINP_FrMCUErr_enum/1 -> Equal1/1, Equal/1
  Constant/1 -> Equal/2
  Equal3/1 -> Logical Operator1/2
  Equal2/1 -> Logical Operator1/1
  Constant3/1 -> Equal3/2
  VINP_RrMCUErr_enum/1 -> Equal3/1, Equal2/1
  Constant2/1 -> Equal2/2
  Logical Operator/1 -> Logical Operator2/1
  Logical Operator1/1 -> Logical Operator2/2

== system tqd/TQD/TorqueDemand/Signal_convert/FWDMCUReadyExt_flg ==
  VINP_FrMCUErr_enum : Inport
  Action Port : ActionPort
  Constant : Constant  Value=ENUM_MCUWARN_LV0
  Constant1 : Constant  Value=ENUM_MCUWARN_NOERROR
  Equal : RelationalOperator  Operator===  OutDataTypeStr=boolean  RndMeth=Simplest
  Equal1 : RelationalOperator  Operator===  OutDataTypeStr=boolean  RndMeth=Simplest
  Logical Operator : Logic  Operator=OR  AllPortsSameDT=off  OutDataTypeStr=boolean
  VTQD_FWDMCUReadyExt_flg : Outport
  wires:
  Logical Operator/1 -> VTQD_FWDMCUReadyExt_flg/1
  Equal/1 -> Logical Operator/1
  VINP_FrMCUErr_enum/1 -> Equal1/1, Equal/1
  Constant/1 -> Equal/2
  Constant1/1 -> Equal1/2
  Equal1/1 -> Logical Operator/2

== system tqd/TQD/TorqueDemand/Signal_convert/New Wheel Slide Rate ==
  VINP_LFRawWhlSpeed_kph : Inport
  VINP_LRRawWhlSpeed_kph : Inport  Port=2
  VINP_RFRawWhlSpeed_kph : Inport  Port=3
  VINP_RRRawWhlSpeed_kph : Inport  Port=4
  VINP_VehSpeed_kph : Inport  Port=5
  task_time_s : Inport  Port=6
  VTQR_NoABSFEDUWhlTqReq_Nm : Inport  Port=7
  VTQR_NoABSREDUWhlTqReq_Nm : Inport  Port=8
  Abs{,1..7} (8 alike) : Abs
  Add : Sum
  Add{1..4} (4 alike) : Sum  Inputs=+-
  Constant{1,4,6,9,11,15,18,135} (8 alike) : Constant  Value=eps
  Constant{5,10,14,128} (4 alike) : Constant  Value=KTQD_NewSlideRateTs_c
  Constant{2,7,12,16,19} (5 alike) : Constant  Value=ZERO_FLOAT
  Constant{3,8,13,17} (4 alike) : Constant  Value=ONE_PERCENT
  Data Type Conversion{,1..3} (4 alike) : DataTypeConversion  OutDataTypeStr=single
  Delay : Delay  DelayLength=1
  Delay1 : Delay  DelayLength=1
  Divide{,1..7} (8 alike) : Product  Inputs=*/
  FirstOrderFilter{,1..3} (4 alike) : hcu_lib/Basic_Blocks/FirstOrderFilter
  Max{,1..3} (4 alike) : MinMax  Function=max  Inputs=2
  Max4 : MinMax  Function=max  Inputs=4
  Max5 : MinMax  Inputs=4
  Min : MinMax  Inputs=5
  Relational Operator{,1..3} (4 alike) : RelationalOperator  Operator=<=  OutDataTypeStr=boolean  RndMeth=Simplest
  Relational Operator{4..7} (4 alike) : RelationalOperator  OutDataTypeStr=boolean  RndMeth=Simplest
  Relational Operator8 : RelationalOperator  Operator=>  OutDataTypeStr=boolean  RndMeth=Simplest
  Switch{,1..8} (9 alike) : Switch  Criteria=u2 > Threshold
  VTQD_MaxWhlSlideRate_pct : Outport
  VTQD_MinWhlSlideRate_pct : Outport  Port=2
  VTQD_LeftSlideRate_pct : Outport  Port=3
  VTQD_RightSlideRate_pct : Outport  Port=4
  VTQD_FrontSlideRate_pct : Outport  Port=5
  VTQD_RearSlideRate_pct : Outport  Port=6
  VTQD_LFSlideRate_pct : Outport  Port=7
  VTQD_LRSlideRate_pct : Outport  Port=8
  VTQD_RFSlideRate_pct : Outport  Port=9
  VTQD_RRSlideRate_pct : Outport  Port=10
  wires:
  [VTQD_RRSlideRate_pct] -> Max4/4
  Divide3/1 -> Switch1/3
  [task_time_s] -> FirstOrderFilter2/2
  [VTQD_FrontSlideRate_pct] -> VTQD_FrontSlideRate_pct/1
  FirstOrderFilter3/1 -> Divide6/1
  Switch4/1 -> [VTQD_LeftSlideRate_pct]  "VTQD_LeftSlideRate_pct"
  Add4/1 -> Divide7/1
  Switch5/1 -> [VTQD_RightSlideRate_pct]  "VTQD_RightSlideRate_pct"
  task_time_s/1 -> [task_time_s]
  [VTQD_LRSlideRate_pct] -> Abs6/1
  FirstOrderFilter1/1 -> Divide2/1
  Divide1/1 -> Switch/3
  Switch6/1 -> [VTQD_FrontSlideRate_pct]  "VTQD_FrontSlideRate_pct"
  Max4/1 -> [VTQD_MaxWhlSlideRate_pct]  "VTQD_MaxWhlSlideRate_pct"
  Constant17/1 -> Divide6/2
  Constant10/1 -> FirstOrderFilter2/3
  [VTQD_LFSlideRate_pct] -> Abs4/1
  Relational Operator4/1 -> Switch4/2
  Max/1 -> Divide1/2
  [VTQD_VehSpeed4Cal_kph] -> Relational Operator3/1
  [VTQD_LRSlideRate_pct] -> Max4/2
  FirstOrderFilter2/1 -> Divide4/1
  Constant13/1 -> Divide4/2
  Divide6/1 -> [VTQD_RRSlideRate_pct]  "VTQD_RRSlideRate_pct"
  Relational Operator6/1 -> Switch6/2
  [VTQD_LFSlideRate_pct] -> Abs/1
  Switch3/1 -> FirstOrderFilter3/1
  [VTQD_LeftSlideRate_pct] -> VTQD_LeftSlideRate_pct/1
  [VTQD_VehSpeed4Cal_kph] -> Max3/1
  [VTQD_RFSlideRate_pct] -> Max5/3
  [VTQD_VehSpeed4Cal_kph] -> Add4/2
  Relational Operator7/1 -> Switch7/2
  Abs5/1 -> Relational Operator6/2
  [task_time_s] -> FirstOrderFilter3/2
  [VINP_RFRawWhlSpeed_kph] -> Add3/1
  Constant14/1 -> FirstOrderFilter3/3
  [VTQD_RRSlideRate_pct] -> Switch7/3
  [task_time_s] -> FirstOrderFilter1/2
  Switch2/1 -> FirstOrderFilter2/1
  Abs6/1 -> Relational Operator7/1
  Constant16/1 -> Switch3/1
  [VTQD_RearSlideRate_pct] -> VTQD_RearSlideRate_pct/1
  Constant18/1 -> Relational Operator3/2
  Max3/1 -> Divide7/2
  Switch7/1 -> [VTQD_RearSlideRate_pct]  "VTQD_RearSlideRate_pct"
  Relational Operator3/1 -> Switch3/2
  [VTQD_LFSlideRate_pct] -> Switch6/1
  Abs/1 -> Relational Operator4/1
  [VTQD_VehSpeed4Cal_kph] -> Relational Operator2/1
  VINP_RFRawWhlSpeed_kph/1 -> [VINP_RFRawWhlSpeed_kph]
  Abs7/1 -> Relational Operator7/2
  Divide/1 -> [VTQD_LFSlideRate_pct]  "VTQD_LFSlideRate_pct"
  [VTQD_RRSlideRate_pct] -> Abs7/1
  Constant2/1 -> Switch/1
  Divide7/1 -> Switch3/3
  [VTQD_LRSlideRate_pct] -> Switch7/1
  Abs1/1 -> Relational Operator4/2
  Relational Operator2/1 -> Switch2/2
  [VTQD_RightSlideRate_pct] -> VTQD_RightSlideRate_pct/1
  [task_time_s] -> FirstOrderFilter/2
  Constant3/1 -> Divide/2
  [VTQD_RFSlideRate_pct] -> Switch6/3
  [VTQD_VehSpeed4Cal_kph] -> Add2/2
  Divide2/1 -> [VTQD_LRSlideRate_pct]  "VTQD_LRSlideRate_pct"
  [VINP_LFRawWhlSpeed_kph] -> Add2/1
  [VTQD_RFSlideRate_pct] -> Abs5/1
  Abs4/1 -> Relational Operator6/1
  VINP_RRRawWhlSpeed_kph/1 -> [VINP_RRRawWhlSpeed_kph]
  Constant9/1 -> Relational Operator2/2
  Constant12/1 -> Switch2/1
  Divide4/1 -> [VTQD_RFSlideRate_pct]  "VTQD_RFSlideRate_pct"
  [VTQD_LRSlideRate_pct] -> Switch4/3
  [VTQD_MinWhlSlideRate_pct] -> VTQD_MinWhlSlideRate_pct/1
  [VTQD_LRSlideRate_pct] -> Max5/2
  [VTQD_RRSlideRate_pct] -> Max5/4
  Max5/1 -> [VTQD_MinWhlSlideRate_pct]  "VTQD_MinWhlSlideRate_pct"
  Constant128/1 -> FirstOrderFilter/3
  [VTQD_LFSlideRate_pct] -> Max5/1
  Abs3/1 -> Relational Operator5/2
  [VTQD_VehSpeed4Cal_kph] -> Max/1
  [VINP_LRRawWhlSpeed_kph] -> Add1/1
  Relational Operator5/1 -> Switch5/2
  [VTQD_RRSlideRate_pct] -> Switch5/3
  [VTQD_RFSlideRate_pct] -> Switch5/1
  Abs2/1 -> Relational Operator5/1
  [VTQD_RRSlideRate_pct] -> Abs3/1
  [VTQD_RFSlideRate_pct] -> Abs2/1
  Constant8/1 -> Divide2/2
  Add2/1 -> Divide1/1
  Constant7/1 -> Switch1/1
  Relational Operator1/1 -> Switch1/2
  Max1/1 -> Divide3/2
  Constant5/1 -> FirstOrderFilter1/3
  Constant4/1 -> Relational Operator1/2
  Switch1/1 -> FirstOrderFilter1/1
  [VTQD_VehSpeed4Cal_kph] -> Relational Operator1/1
  [VTQD_VehSpeed4Cal_kph] -> Max1/1
  Add1/1 -> Divide3/1
  [VTQD_VehSpeed4Cal_kph] -> Add1/2
  VINP_LFRawWhlSpeed_kph/1 -> [VINP_LFRawWhlSpeed_kph]
  Relational Operator/1 -> Switch/2
  [VTQD_VehSpeed4Cal_kph] -> Relational Operator/1
  Constant1/1 -> Relational Operator/2
  [VTQD_LRSlideRate_pct] -> Abs1/1
  VINP_VehSpeed_kph/1 -> [VINP_VehSpeed_kph]
  VINP_LRRawWhlSpeed_kph/1 -> [VINP_LRRawWhlSpeed_kph]
  [VTQD_RFSlideRate_pct] -> Max4/3
  [VTQD_MaxWhlSlideRate_pct] -> VTQD_MaxWhlSlideRate_pct/1
  [VINP_RRRawWhlSpeed_kph] -> Add4/1
  FirstOrderFilter/1 -> Divide/1
  Switch/1 -> FirstOrderFilter/1
  [VTQD_LFSlideRate_pct] -> Switch4/1
  [VTQD_LFSlideRate_pct] -> Max4/1
  [VTQD_VehSpeed4Cal_kph] -> Add3/2
  [VTQD_VehSpeed4Cal_kph] -> Max2/1
  Add3/1 -> Divide5/1
  Max2/1 -> Divide5/2
  Divide5/1 -> Switch2/3
  Constant11/1 -> Data Type Conversion/1
  Data Type Conversion/1 -> Max2/2
  Data Type Conversion1/1 -> Max1/2
  Constant6/1 -> Data Type Conversion1/1
  Data Type Conversion2/1 -> Max/2
  Constant135/1 -> Data Type Conversion2/1
  Data Type Conversion3/1 -> Max3/2
  Constant15/1 -> Data Type Conversion3/1
  VTQR_NoABSFEDUWhlTqReq_Nm/1 -> [VTQR_NoABSFEDUWhlTqReq_Nm]
  VTQR_NoABSREDUWhlTqReq_Nm/1 -> [VTQR_NoABSREDUWhlTqReq_Nm]
  Add/1 -> Relational Operator8/1
  [VINP_VehSpeed_kph] -> Switch8/3
  Constant19/1 -> Relational Operator8/2
  Relational Operator8/1 -> Switch8/2
  Min/1 -> Switch8/1
  [VINP_LFRawWhlSpeed_kph] -> Min/1
  [VINP_LRRawWhlSpeed_kph] -> Min/2
  [VINP_RFRawWhlSpeed_kph] -> Min/3
  [VINP_RRRawWhlSpeed_kph] -> Min/4
  [VINP_VehSpeed_kph] -> Min/5
  [VTQR_NoABSFEDUWhlTqReq_Nm] -> Delay/1
  Delay/1 -> Add/1
  Delay1/1 -> Add/2
  [VTQR_NoABSREDUWhlTqReq_Nm] -> Delay1/1
  Switch8/1 -> [VTQD_VehSpeed4Cal_kph]  "VTQD_VehSpeed4Cal_kph"
  [VTQD_LRSlideRate_pct] -> VTQD_LRSlideRate_pct/1
  [VTQD_RRSlideRate_pct] -> VTQD_RRSlideRate_pct/1
  [VTQD_LFSlideRate_pct] -> VTQD_LFSlideRate_pct/1
  [VTQD_RFSlideRate_pct] -> VTQD_RFSlideRate_pct/1

== system tqd/TQD/TorqueDemand/Signal_convert/OUTPUT ONLY ON or READY ==
  note: INPUT Signals
  VPMM_PowerSta_enum : Inport
  VTQD_SWCRegenUpSta_flg : Inport  Port=2
  VTQD_SWCRegenDownSta_flg : Inport  Port=3
  VINP_ADASACCSta_enum : Inport  Port=4
  VVMC_CCCtrlSta_enum : Inport  Port=5
  VBCM_BrakeLamp_flg : Inport  Port=6
  VINP_VehSpeed_kph : Inport  Port=7
  AND : Logic  Inputs=6  AllPortsSameDT=off  OutDataTypeStr=boolean
  Constant1 : Constant  Value=ENUM_ADASACCSTA_ACTIVE
  Constant10 : Constant  Value=FALSE
  Constant11 : Constant  Value=KTQD_RegenButEnSpd_kph
  Constant3 : Constant  Value=ENUM_POWERSTA_ON
  Constant5 : Constant  Value=FALSE
  Constant6 : Constant  Value=ENUM_ADASACCSTA_OVERRIDE
  Constant7 : Constant  Value=ENUM_POWERSTA_READY
  Constant8 : Constant  Value=ENUM_ADASCCSTA_ACTIVE
  Constant9 : Constant  Value=ENUM_ADASCCSTA_OVRRIDE
  Equal2 : RelationalOperator  Operator===  OutDataTypeStr=boolean  RndMeth=Simplest
  Equal3 : RelationalOperator  Operator===  OutDataTypeStr=boolean  RndMeth=Simplest
  Equal{4..7} (4 alike) : RelationalOperator  Operator=~=  OutDataTypeStr=boolean  RndMeth=Simplest
  NOT : Logic  Operator=NOT  AllPortsSameDT=off  OutDataTypeStr=boolean
  OR1 : Logic  Operator=OR  AllPortsSameDT=off  OutDataTypeStr=boolean
  OR2 : Logic  Operator=OR  AllPortsSameDT=off  OutDataTypeStr=boolean
  Relational Operator : RelationalOperator  Operator=<=  OutDataTypeStr=boolean  RndMeth=Simplest
  Switch : Switch  Criteria=u2 ~= 0
  Switch1 : Switch  Criteria=u2 ~= 0
  SWC_RegenUp : Outport
  SWC_RegenDown : Outport  Port=2
  wires:
  Constant5/1 -> Switch/3
  Switch/1 -> SWC_RegenUp/1  "SWC_RegenUp"
  VTQD_SWCRegenUpSta_flg/1 -> Switch/1
  VTQD_SWCRegenDownSta_flg/1 -> Switch1/1
  Switch1/1 -> SWC_RegenDown/1  "SWC_RegenDown"
  Constant10/1 -> Switch1/3
  AND/1 -> Switch1/2, Switch/2
  VPMM_PowerSta_enum/1 -> [VPMM_PowerSta_enum]
  VINP_ADASACCSta_enum/1 -> [VINP_ADASACCSta_enum]
  VVMC_CCCtrlSta_enum/1 -> [VVMC_CCCtrlSta_enum]
  VBCM_BrakeLamp_flg/1 -> [VBCM_BrakeLamp_flg]
  VINP_VehSpeed_kph/1 -> [VINP_VehSpeed_kph]
  Relational Operator/1 -> OR2/2
  NOT/1 -> OR2/1
  OR2/1 -> AND/6
  Constant11/1 -> Relational Operator/2
  [VINP_VehSpeed_kph] -> Relational Operator/1
  Equal4/1 -> AND/2
  Equal5/1 -> AND/3
  Equal6/1 -> AND/4
  Equal7/1 -> AND/5
  OR1/1 -> AND/1
  Constant8/1 -> Equal6/2
  Constant9/1 -> Equal7/2
  [VBCM_BrakeLamp_flg] -> NOT/1
  [VVMC_CCCtrlSta_enum] -> Equal7/1
  [VVMC_CCCtrlSta_enum] -> Equal6/1
  [VINP_ADASACCSta_enum] -> Equal5/1
  Constant6/1 -> Equal5/2
  Constant1/1 -> Equal4/2
  [VINP_ADASACCSta_enum] -> Equal4/1
  Equal3/1 -> OR1/2
  [VPMM_PowerSta_enum] -> Equal2/1
  Constant7/1 -> Equal3/2
  Constant3/1 -> Equal2/2
  Equal2/1 -> OR1/1
  [VPMM_PowerSta_enum] -> Equal3/1

== system tqd/TQD/TorqueDemand/Signal_convert/RWDMCUReadyExt_flg ==
  VINP_RrMCUErr_enum : Inport
  Action Port : ActionPort
  Constant : Constant  Value=ENUM_MCUWARN_LV0
  Constant1 : Constant  Value=ENUM_MCUWARN_NOERROR
  Equal : RelationalOperator  Operator===  OutDataTypeStr=boolean  RndMeth=Simplest
  Equal1 : RelationalOperator  Operator===  OutDataTypeStr=boolean  RndMeth=Simplest
  Logical Operator : Logic  Operator=OR  AllPortsSameDT=off  OutDataTypeStr=boolean
  VTQD_RWDMCUReadyExt_flg : Outport
  wires:
  Logical Operator/1 -> VTQD_RWDMCUReadyExt_flg/1
  VINP_RrMCUErr_enum/1 -> Equal1/1, Equal/1
  Equal1/1 -> Logical Operator/2
  Equal/1 -> Logical Operator/1
  Constant1/1 -> Equal1/2
  Constant/1 -> Equal/2

== system tqd/TQD/TorqueDemand/Signal_convert/Regen Level Switch Botton ==
  task_time_s : Inport
  SWC_RegenUp : Inport  Port=2
  SWC_RegenDown : Inport  Port=3
  Constant13 : Constant  Value=ENUM_REGENSWSTA_SHORTPRESSUP
  Constant18 : Constant  Value=ENUM_REGENSWSTA_LONGPRESSUP
  Constant21 : Constant  Value=ENUM_REGENSWSTA_SHORTPRESSDOWN
  Constant23 : Constant  Value=ENUM_REGENSWSTA_LONGPRESSDOWN
  Constant24 : Constant  Value=ENUM_REGENSWSTA_NOACTION
  RegenDOWN : Subsystem
  RegenUP : Subsystem
  Switch{4,6..8} (4 alike) : Switch  Criteria=u2 ~= 0
  VTQD_RegenSWSta_enum : Outport
  wires:
  [SWC_RegenUP] -> RegenUP/2(SWC_RegenUp)
  Constant24/1 -> Switch8/3
  Constant13/1 -> Switch4/1
  [SWC_RegenDown] -> RegenDOWN/3(SWC_RegenDOWN)
  RegenDOWN/2(VTQD_RegenDownLongP_flg) -> Switch8/2
  Constant23/1 -> Switch8/1
  Constant21/1 -> Switch7/1
  Switch7/1 -> Switch6/3
  RegenDOWN/1(SWC_RegenDownShort_flg) -> Switch7/2
  [SWC_RegenUP] -> RegenDOWN/2(SWC_RegenUp)
  Constant18/1 -> Switch6/1
  RegenUP/2(VTQD_RegenUpLongP_flg) -> Switch6/2
  Switch6/1 -> Switch4/3
  RegenUP/1(SWC_RegenUpShort_flg) -> Switch4/2
  [SWC_RegenDown] -> RegenUP/3(SWC_RegenDOWN)
  SWC_RegenUp/1 -> [SWC_RegenUP]
  SWC_RegenDown/1 -> [SWC_RegenDown]
  Switch8/1 -> Switch7/3
  Switch4/1 -> VTQD_RegenSWSta_enum/1
  task_time_s/1 -> [task_time_s]
  [task_time_s] -> RegenUP/1(task_time_s)
  [task_time_s] -> RegenDOWN/1(task_time_s)
